simulink model "base_model_2020b_WS2223"  (R2022b)
settings: Solver=FixedStepDiscrete  StartTime=0.0  StopTime=10  FixedStep=0.01  RelTol=1e-3
libraries: simulink x4
settings Model: Creator=paulplusx  LastModifiedBy=erikd
settings SolverCC: AlgebraicLoopSolver=TrustRegion
settings DebuggingCC: UnconnectedInputMsg=warning  UnconnectedOutputMsg=warning  UnconnectedLineMsg=warning  SFMachineParentedDataDiag=warning
settings ModelReferenceCC: EnableRefExpFcnMdlSchedulingChecks=on
settings RTWCC: DLArmComputeVersion=19.05

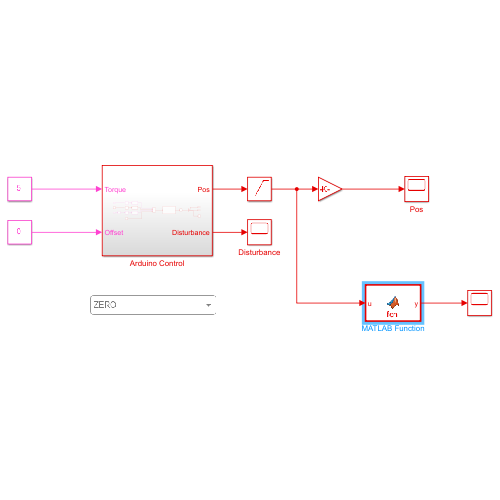
[thumbnail: Simulink's stored preview of the top-level diagram]
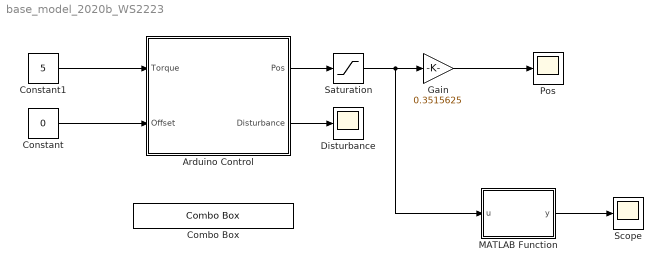
== system base_model_2020b_WS2223 ==
  Arduino Control : Subsystem
  Combo Box : ComboBox  LabelPosition=Hide  SelectedLabel=ZERO
      settings: Values={{'ZERO', 'TYPE1', 'TYPE2', 'TYPE3', 'TYPE4', 'TYPE5', 'TYPE6', 'TYPE7', 'TYPE8', 'TYPE9'}, [0 1 2 3 4 5 6 7 8 9]}
  Constant : Constant  Value=0  OutDataTypeStr=int32
  Constant1 : Constant  Value=5  OutDataTypeStr=int32  SampleTime=Inf
  Disturbance : Scope
  Gain : Gain  Gain=0.3515625
  MATLAB Function : MATLAB Function  TreatAsAtomicUnit=on
  Pos : Scope
  Saturation : Saturate  UpperLimit=1024  LowerLimit=0
  Scope : Scope
  wires:
  Constant1/1 -> Arduino Control/1(Torque)
  Arduino Control/2(Disturbance) -> Disturbance/1
  Constant/1 -> Arduino Control/2(Offset)
  Gain/1 -> Pos/1
  Arduino Control/1(Pos) -> Saturation/1
  Saturation/1 -> MATLAB Function/1(u), Gain/1
  MATLAB Function/1(y) -> Scope/1

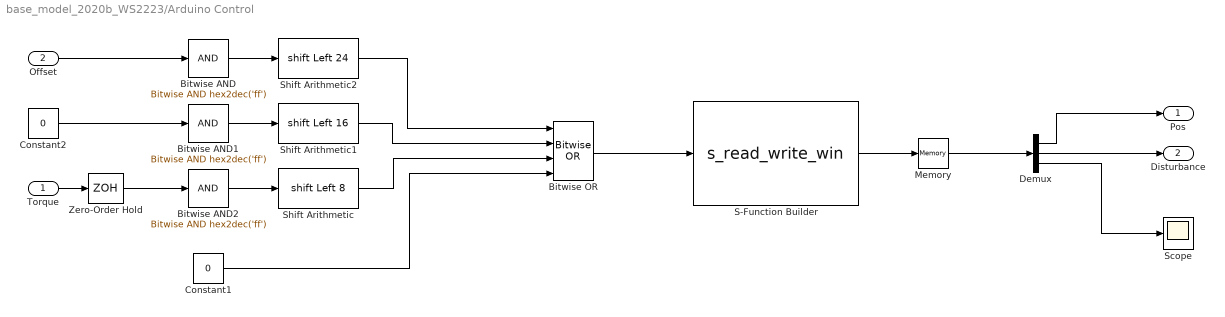
== system base_model_2020b_WS2223/Arduino Control ==
  Torque : Inport
  Offset : Inport  Port=2
  Bitwise AND : simulink/Logic and Bit Operations/Bitwise Operator  logicop=AND  UseBitMask=on  BitMask=hex2dec('ff')  BitMaskRealWorld=Stored Integer
  Bitwise AND1 : simulink/Logic and Bit Operations/Bitwise Operator  logicop=AND  UseBitMask=on  BitMask=hex2dec('ff')  BitMaskRealWorld=Stored Integer
  Bitwise AND2 : simulink/Logic and Bit Operations/Bitwise Operator  logicop=AND  UseBitMask=on  BitMask=hex2dec('ff')  BitMaskRealWorld=Stored Integer
  Bitwise OR : simulink/Logic and Bit Operations/Bitwise Operator  logicop=OR  UseBitMask=off  NumInputPorts=4  BitMask=bin2dec('11011001')  BitMaskRealWorld=Stored Integer
  Constant1 : Constant  Value=0  OutDataTypeStr=int32  SampleTime=-1
  Constant2 : Constant  Value=0  OutDataTypeStr=int32  SampleTime=-1
  Demux : Demux  Outputs=3
  Memory : Memory
  S-Function Builder : S-Function  FunctionName=s_read_write_win  SFunctionModules=s_read_write_win_wrapper  SFunctionDeploymentMode=off  EnableBusSupport=off  mask(S-Function Builder){}
      mask help: Simulink:masks:SFunctionBuilder_MD
      mask init:
      | val = [[.9  0.75 0.75 1 1 .9 .9 1]',[1 1 0.75 0.75 .9 .9 1 .9]'];try , sys = get_param(gcb,'SfunBuilderFcnName');if isempty(sys), sys = get_param(gcb,'FunctionName'); end,catch, sys = get_param(gcb,'FunctionName'); end
      settings: CopyFcn=set_param(gcbh,'LinkStatus','none')  OpenFcn=sfunctionwizard(gcbh)
      mask Display:
      | plot(val(:,1),val(:,2))
      | disp(sys)
      | port_label('input',1,'TX')
      | port_label('output',1,'RX')
  Scope : Scope
  Shift Arithmetic : ArithShift  BitShiftNumber=8  BitShiftDirection=Left
  Shift Arithmetic1 : ArithShift  BitShiftNumber=16  BitShiftDirection=Left
  Shift Arithmetic2 : ArithShift  BitShiftNumber=24  BitShiftDirection=Left
  Zero-Order Hold : ZeroOrderHold  SampleTime=-1
  Pos : Outport
  Disturbance : Outport  Port=2
  wires:
  Shift Arithmetic2/1 -> Bitwise OR/1
  Zero-Order Hold/1 -> Bitwise AND2/1
  Bitwise AND2/1 -> Shift Arithmetic/1
  Shift Arithmetic1/1 -> Bitwise OR/2
  Bitwise AND/1 -> Shift Arithmetic2/1
  Bitwise OR/1 -> S-Function Builder/1
  Bitwise AND1/1 -> Shift Arithmetic1/1
  Shift Arithmetic/1 -> Bitwise OR/3
  Memory/1 -> Demux/1
  S-Function Builder/1 -> Memory/1
  Constant2/1 -> Bitwise AND1/1
  Offset/1 -> Bitwise AND/1
  Torque/1 -> Zero-Order Hold/1
  Constant1/1 -> Bitwise OR/4
  Demux/1 -> Pos/1
  Demux/2 -> Disturbance/1
  Demux/3 -> Scope/1

== matlab function base_model_2020b_WS2223/MATLAB Function ==
  data: u input; y output
function y = fcn(u)

y = 360.0/1024.0 * u;
